simulink library "outp"  (R2021b)
(part 3 of 11)

  bus_selector3/179 -> outpmodule/357(VBCM_WinRROpenedSta_pct)  "<VBCM_WinRROpenedSta_pct>"
  bus_selector13/31 -> outpmodule/953(VTQD_FrUdcMin_V)  "<VTQD_FrUdcMin_V>"
  bus_selector2/16 -> outpmodule/19(VAPM_APSDFLR_cm)  "<VAPM_APSDFLR_cm>"
  outpmodule/782(VOUTP_FDCTHCCREVentZStaSet7_enum) -> bus_creator/782
  bus_selector12/68 -> outpmodule/893(VTPM_ChkStorge_flg)  "<VTPM_ChkStorge_flg>"
  bus_selector3/175 -> outpmodule/353(VBCM_CLWinLockDrStaMem_enum)  "<VBCM_CLWinLockDrStaMem_enum>"
  outpmodule/248(VOUTP_IVIRST_flg) -> bus_creator/248
  bus_selector16/7 -> outpmodule/989(VVMC_VMCCCCtrlAvail_flg)  "<VVMC_VMCCCCtrlAvail_flg>"
  outpmodule/644(VOUTP_ECUGen2_cnt) -> bus_creator/644
  bus_selector11/129 -> outpmodule/778(VTHC_FDCTHCCREVentZStaSet2_enum)  "<VTHC_FDCTHCCREVentZStaSet2_enum>"
  outpmodule/706(VOUTP_FDCTHCREVentZSta_enum) -> bus_creator/706
  bus_selector3/173 -> outpmodule/351(VBCM_PsRWdwReqAP_enum)  "<VBCM_PsRWdwReqAP_enum>"
  bus_selector3/171 -> outpmodule/349(VBCM_PasWdwReqAP_enum)  "<VBCM_PasWdwReqAP_enum>"
  outpmodule/832(VOUTP_LRWheelPress_raw8) -> bus_creator/832
  bus_selector10/35 -> outpmodule/641(VSYS_AcoreRebootCmdACK_flg)  "<VSYS_AcoreRebootCmdACK_flg>"
  bus_selector13/39 -> outpmodule/961(VTQD_EquivAccPedalSWSta_flg)  "<VTQD_EquivAccPedalSWSta_flg>"
  bus_selector3/172 -> outpmodule/350(VBCM_DrRWdwReqAP_enum)  "<VBCM_DrRWdwReqAP_enum>"
  outpmodule/1044(VOUTP_LKAHODDisplayWarning_flg) -> bus_creator/1044
  bus_selector3/170 -> outpmodule/348(VBCM_DrvWdwReqAP_enum)  "<VBCM_DrvWdwReqAP_enum>"
  outpmodule/714(VOUTP_FDCTHCCREVentYSta_enum) -> bus_creator/714
  outpmodule/236(VOUTP_AmbLightBrightness5_enum) -> bus_creator/236
  outpmodule/799(VOUTP_FDCTHCREVentYStaSet5_enum) -> bus_creator/799
  bus_selector3/168 -> outpmodule/346(VBCM_HMIKey8FuncSta_enum)  "<VBCM_HMIKey8FuncSta_enum>"
  bus_selector3/164 -> outpmodule/342(VBCM_HMIKey4FuncSta_enum)  "<VBCM_HMIKey4FuncSta_enum>"
  bus_selector3/165 -> outpmodule/343(VBCM_HMIKey5FuncSta_enum)  "<VBCM_HMIKey5FuncSta_enum>"
  bus_selector3/166 -> outpmodule/344(VBCM_HMIKey6FuncSta_enum)  "<VBCM_HMIKey6FuncSta_enum>"
  outpmodule/1032(VOUTP_RightTurnLightReq_flg) -> bus_creator/1032
  outpmodule/937(VOUTP_FrEDUActTq_Nm) -> bus_creator/937
  outpmodule/178(VOUTP_IVIUserTakeOverAPSSta_flg) -> bus_creator/178
  bus_selector10/3 -> outpmodule/609(VSYS_HWVer3_cnt)  "<VSYS_HWVer3_cnt>"
  bus_selector16/12 -> outpmodule/994(VVMC_LimitPCT_pct)  "<VVMC_LimitPCT_pct>"
  bus_selector3/163 -> outpmodule/341(VBCM_HMIKey3FuncSta_enum)  "<VBCM_HMIKey3FuncSta_enum>"
  outpmodule/788(VOUTP_FDCTHCLEVentYStaSet7_enum) -> bus_creator/788
  bus_selector6/10 -> outpmodule/534(VDKC_DKeyWelcomeSta_enum)  "<VDKC_DKeyWelcomeSta_enum>"
  outpmodule/98(VOUTP_SASSpeedValidTimeOut_flg) -> bus_creator/98
  outpmodule/611(VOUTP_CarModel2_cnt) -> bus_creator/611
  outpmodule/980(VOUTP_ReqOBCIntrV2LEna_enum) -> bus_creator/980
  bus_selector3/158 -> outpmodule/336(VBCM_AutoLockMem_enum)  "<VBCM_AutoLockMem_enum>"
  bus_selector3/160 -> outpmodule/338(VBCM_AutoUnlockMem_enum)  "<VBCM_AutoUnlockMem_enum>"
  outpmodule/892(VOUTP_TPMSStorge_flg) -> bus_creator/892
  bus_selector10/42 -> outpmodule/648(VSYS_Var4_cnt)  "<VSYS_Var4_cnt>"
  outpmodule/491(VOUTP_EngagePFail_flg) -> bus_creator/491
  bus_selector3/157 -> outpmodule/335(VBCM_AutoLockSta_flg)  "<VBCM_AutoLockSta_flg>"
  bus_selector4/138 -> outpmodule/495(VDDM_EDriveSysErrShifterErr_flg)  "<VDDM_EDriveSysErrShifterErr_flg>"
  bus_selector11/83 -> outpmodule/732(VTHC_sigRecircStSet_enum)  "<VTHC_sigRecircStSet_enum>"
  bus_selector3/155 -> outpmodule/333(VBCM_LRightStaCmd_flg)  "<VBCM_LRightStaCmd_flg>"
  outpmodule/999(VOUTP_SafetyCtrl_flg) -> bus_creator/999
  bus_selector3/73 -> outpmodule/251(VBCM_MirrorFlodPos_flg)  "<VBCM_MirrorFlodPos_flg>"
  bus_selector13/25 -> outpmodule/947(VTQD_RgnAbnorSta_flg)  "<VTQD_RgnAbnorSta_flg>"
  bus_selector3/161 -> outpmodule/339(VBCM_HMIKey1FuncSta_enum)  "<VBCM_HMIKey1FuncSta_enum>"
  bus_selector12/72 -> outpmodule/897(VTPM_LRPindi_enum)  "<VTPM_LRPindi_enum>"
  bus_selector4/145 -> outpmodule/502(VDDM_VCURLDoorSta_flg)  "<VDDM_VCURLDoorSta_flg>"
  bus_selector2/166 -> outpmodule/169(VAPM_CAASVMCReqA_flg)  "<VAPM_CAASVMCReqA_flg>"
  bus_selector11/20 -> outpmodule/669(VTHC_BatteryMode_enum)  "<VTHC_BatteryMode_enum>"
  bus_selector3/150 -> outpmodule/328(VBCM_SenstivityPosnCmd_enum)  "<VBCM_SenstivityPosnCmd_enum>"
  outpmodule/617(VOUTP_Minor1_cnt) -> bus_creator/617
  outpmodule/225(VOUTP_WiperFixMode_flg) -> bus_creator/225
  bus_selector9/11 -> outpmodule/569(VPMM_LVPwrSta_flg)  "<VPMM_LVPwrSta_flg>"
  outpmodule/906(VOUTP_WriteChkfinRRID_raw) -> bus_creator/906
  outpmodule/228(VOUTP_AmbLightBreath3_enum) -> bus_creator/228
  bus_selector3/151 -> outpmodule/329(VBCM_TimeGapLevelSta_enum)  "<VBCM_TimeGapLevelSta_enum>"
  outpmodule/993(VOUTP_JerkPCT_pct) -> bus_creator/993
  bus_selector3/148 -> outpmodule/326(VBCM_PTGOpenHeight34_enum)  "<VBCM_PTGOpenHeight34_enum>"
  bus_selector2/24 -> outpmodule/27(VAPM_PASAFML_enum)  "<VAPM_PASAFML_enum>"
  bus_selector3/149 -> outpmodule/327(VBCM_PTGOpenHeight57_enum)  "<VBCM_PTGOpenHeight57_enum>"
  outpmodule/689(VOUTP_ACModeMem_enum) -> bus_creator/689
  bus_selector3/146 -> outpmodule/324(VBCM_PTGUserHeight7_cnt)  "<VBCM_PTGUserHeight7_cnt>"
  bus_selector11/36 -> outpmodule/685(VTHC_sigAmbAirT_C)  "<VTHC_sigAmbAirT_C>"
  bus_selector11/106 -> outpmodule/755(VTHC_LEVentModeStaSet123_enum)  "<VTHC_LEVentModeStaSet123_enum>"
  bus_selector3/78 -> outpmodule/256(VBCM_PasWdwCtrlCmd_pct)  "<VBCM_PasWdwCtrlCmd_pct>"
  outpmodule/187(VOUTP_DrDoorSW_flg) -> bus_creator/187
  outpmodule/1002(VOUTP_ISOAccLimit_mps2) -> bus_creator/1002
  bus_selector3/145 -> outpmodule/323(VBCM_PTGUserHeight5_cnt)  "<VBCM_PTGUserHeight5_cnt>"
  bus_selector2/79 -> outpmodule/82(VAPM_RFPulseCountTimeOut_flg)  "<VAPM_RFPulseCountTimeOut_flg>"
  bus_selector12/2 -> outpmodule/827(VTPM_RFBatWarn_flg)  "<VTPM_RFBatWarn_flg>"
  bus_selector3/143 -> outpmodule/321(VBCM_PTGUserHeight3_cnt)  "<VBCM_PTGUserHeight3_cnt>"
  bus_selector3/144 -> outpmodule/322(VBCM_PTGUserHeight4_cnt)  "<VBCM_PTGUserHeight4_cnt>"
  bus_selector4/118 -> outpmodule/475(VDDM_RRPressIndiDTC_raw32)  "<VDDM_RRPressIndiDTC_raw32>"
  bus_selector3/15 -> outpmodule/193(VBCM_RrChargingDoorCtrl_enum)  "<VBCM_RrChargingDoorCtrl_enum>"
  bus_selector3/13 -> outpmodule/191(VBCM_LockSetting_flg)  "<VBCM_LockSetting_flg>"
  outpmodule/231(VOUTP_AmbLightBreath6_enum) -> bus_creator/231
  bus_selector2/4 -> outpmodule/7(VAPM_FSOffSwTimeOut_flg)  "<VAPM_FSOffSwTimeOut_flg>"
  bus_selector3/12 -> outpmodule/190(VBCM_RRDoorSW_flg)  "<VBCM_RRDoorSW_flg>"
  outpmodule/736(VOUTP_AirIntenZone1MSet3_enum) -> bus_creator/736
  outpmodule/914(VOUTP_FlashS3ID_raw) -> bus_creator/914
  bus_selector3/11 -> outpmodule/189(VBCM_RLDoorSW_flg)  "<VBCM_RLDoorSW_flg>"
  bus_selector3/8 -> outpmodule/186(VBCM_TailgateSW_flg)  "<VBCM_TailgateSW_flg>"
  bus_selector3/35 -> outpmodule/213(VBCM_BCMBuzzerReq_flg)  "<VBCM_BCMBuzzerReq_flg>"
  bus_selector2/111 -> outpmodule/114(VAPM_YawRateVTimeOut_flg)  "<VAPM_YawRateVTimeOut_flg>"
  bus_selector3/10 -> outpmodule/188(VBCM_PsDoorSW_flg)  "<VBCM_PsDoorSW_flg>"
  outpmodule/868(VOUTP_S2ID_raw32) -> bus_creator/868
  outpmodule/81(VOUTP_RFPulseCount_enum) -> bus_creator/81
  outpmodule/84(VOUTP_LRPulseCountTimeOut_flg) -> bus_creator/84
  outpmodule/241(VOUTP_AmbLightColor4_enum) -> bus_creator/241
  outpmodule/1028(VOUTP_ADASShftPosnReqA_flg) -> bus_creator/1028
  outpmodule/442(VOUTP_FCM5CSErrDTC_raw32) -> bus_creator/442
  bus_selector16/22 -> outpmodule/1004(VVMC_ISOJerkLimit_mps3)  "<VVMC_ISOJerkLimit_mps3>"
  outpmodule/724(VOUTP_FDCTHCMPreWPTCHeatSta_enum) -> bus_creator/724
  bus_selector2/125 -> outpmodule/128(VAPM_ESCAPSStaTimeOut_flg)  "<VAPM_ESCAPSStaTimeOut_flg>"
  outpmodule/673(VOUTP_CCUAutoLampSts_flg) -> bus_creator/673
  outpmodule/249(VOUTP_CountAlarm_enum) -> bus_creator/249
  bus_selector9/35 -> outpmodule/593(VPMM_LVSilentChrgReq_flg)  "<VPMM_LVSilentChrgReq_flg>"
  outpmodule/118(VOUTP_LongAccelVTimeOut_flg) -> bus_creator/118
  outpmodule/777(VOUTP_FDCTHCCREVentZStaSet1_enum) -> bus_creator/777
  bus_selector2/126 -> outpmodule/129(VAPM_EPBExtReleaseAvail_flg)  "<VAPM_EPBExtReleaseAvail_flg>"
  outpmodule/701(VOUTP_FDCTHCAirIntZ3Sta_enum) -> bus_creator/701
  bus_selector2/124 -> outpmodule/127(VAPM_ESCAPSSta_enum)  "<VAPM_ESCAPSSta_enum>"
  bus_selector9/26 -> outpmodule/584(VPMM_PwrStaONTOPopReq_flg)  "<VPMM_PwrStaONTOPopReq_flg>"
  bus_selector2/137 -> outpmodule/140(VAPM_AVMparkingexcuteTimeOut_flg)  "<VAPM_AVMparkingexcuteTimeOut_flg>"
  bus_selector3/113 -> outpmodule/291(VBCM_DimSwSta_flg)  "<VBCM_DimSwSta_flg>"
  bus_selector3/177 -> outpmodule/355(VBCM_WinRFOpenedSta_pct)  "<VBCM_WinRFOpenedSta_pct>"
  bus_selector4/46 -> outpmodule/403(VDDM_TailgaSWDTC_raw32)  "<VDDM_TailgaSWDTC_raw32>"
  bus_selector11/120 -> outpmodule/769(VTHC_FDCTHCCLEVentZStaSet5_enum)  "<VTHC_FDCTHCCLEVentZStaSet5_enum>"
  bus_selector3/55 -> outpmodule/233(VBCM_AmbLightBrightness2_enum)  "<VBCM_AmbLightBrightness2_enum>"
  bus_selector2/132 -> outpmodule/135(VAPM_EPBSta_enum)  "<VAPM_EPBSta_enum>"
  bus_selector2/131 -> outpmodule/134(VAPM_EPBErrStaTimeOut_flg)  "<VAPM_EPBErrStaTimeOut_flg>"
  bus_selector4/34 -> outpmodule/391(VDDM_HVRlyOpDTC_raw32)  "<VDDM_HVRlyOpDTC_raw32>"
  bus_selector6/13 -> outpmodule/537(VDKC_UIDLowPowerSta_enum)  "<VDKC_UIDLowPowerSta_enum>"
  bus_selector11/175 -> outpmodule/824(VTHC_THSysErrlampReq_flg)  "<VTHC_THSysErrlampReq_flg>"
  bus_selector6/2 -> outpmodule/526(VDKC_DKCAuthSta_enum)  "<VDKC_DKCAuthSta_enum>"
  bus_selector4/38 -> outpmodule/395(VDDM_LVSupLoDTC_raw32)  "<VDDM_LVSupLoDTC_raw32>"
  outpmodule/56(VOUTP_LFRawWhlSpeedVTimeOut_flg) -> bus_creator/56
  bus_selector11/18 -> outpmodule/667(VTHC_FDRrAPTCHeatPwrCmd_W)  "<VTHC_FDRrAPTCHeatPwrCmd_W>"
  outpmodule/54(VOUTP_RRRawWhlSpeedTimeOut_flg) -> bus_creator/54
  outpmodule/911(VOUTP_Prepresstempvalid_enum) -> bus_creator/911
  outpmodule/217(VOUTP_RoomLampH_flg) -> bus_creator/217
  bus_selector2/162 -> outpmodule/165(VAPM_CAASSta_enum)  "<VAPM_CAASSta_enum>"
  bus_selector11/166 -> outpmodule/815(VTHC_FACESet_enum)  "<VTHC_FACESet_enum>"
  bus_selector3/28 -> outpmodule/206(VBCM_LDRL_flg)  "<VBCM_LDRL_flg>"
  outpmodule/55(VOUTP_LFRawWhlSpeedV_flg) -> bus_creator/55
  outpmodule/252(VOUTP_FuelDoorPos_flg) -> bus_creator/252
  bus_selector11/113 -> outpmodule/762(VTHC_FDCTHCLEVentZStaSet4_enum)  "<VTHC_FDCTHCLEVentZStaSet4_enum>"
  outpmodule/53(VOUTP_RRRawWhlSpeed_kph) -> bus_creator/53
  outpmodule/49(VOUTP_RFRawWhlSpeed_kph) -> bus_creator/49
  outpmodule/641(VOUTP_AcoreRebootCmdACK_flg) -> bus_creator/641
  outpmodule/95(VOUTP_SASSpeed_degps) -> bus_creator/95
  bus_selector2/158 -> outpmodule/161(VAPM_APSExitCondition_enum)  "<VAPM_APSExitCondition_enum>"
  outpmodule/50(VOUTP_RFRawWhlSpeedTimeOut_flg) -> bus_creator/50
  outpmodule/921(VOUTP_ModelVersion_raw) -> bus_creator/921
  outpmodule/734(VOUTP_AirIntenZone1MSet1_enum) -> bus_creator/734
  bus_selector9/23 -> outpmodule/581(VPMM_LowSOCWarn_enum)  "<VPMM_LowSOCWarn_enum>"
  outpmodule/308(VOUTP_RmLpModeENMem_enum) -> bus_creator/308
  outpmodule/48(VOUTP_LFRawWhlSpeedTimeOut_flg) -> bus_creator/48
  outpmodule/1061(VOUTP_ADASLanetypeR_enum) -> bus_creator/1061
  outpmodule/988(VOUTP_VMCACCCtrlAvail_flg) -> bus_creator/988
  bus_selector3/114 -> outpmodule/292(VBCM_PassSWSta_flg)  "<VBCM_PassSWSta_flg>"
  bus_selector4/43 -> outpmodule/400(VDDM_FRDoorSWDTC_raw32)  "<VDDM_FRDoorSWDTC_raw32>"
  outpmodule/524(VOUTP_EAPS2NRM_pct) -> bus_creator/524
  outpmodule/505(VOUTP_VCUHoodSWSta_flg) -> bus_creator/505
  outpmodule/46(VOUTP_BrkPedalPosTimeOut_flg) -> bus_creator/46
  bus_selector11/54 -> outpmodule/703(VTHC_FDCTHCREVentModeSta_enum)  "<VTHC_FDCTHCREVentModeSta_enum>"
  outpmodule/44(VOUTP_ModOperation_enum) -> bus_creator/44
  outpmodule/915(VOUTP_FlashS4ID_raw) -> bus_creator/915
  outpmodule/575(VOUTP_DrSeatSta_enum) -> bus_creator/575
  bus_selector14/1 -> outpmodule/974(VTQR_FrTMTqReq_Nm)  "<VTQR_FrTMTqReq_Nm>"
  outpmodule/42(VOUTP_SNSRLayout_enum) -> bus_creator/42
  outpmodule/262(VOUTP_AmbDimEN_flg) -> bus_creator/262
  outpmodule/40(VOUTP_USSStaFCL_flg) -> bus_creator/40
  bus_selector2/90 -> outpmodule/93(VAPM_SASAngle_Deg)  "<VAPM_SASAngle_Deg>"
  bus_selector3/82 -> outpmodule/260(VBCM_AmbFunEN_flg)  "<VBCM_AmbFunEN_flg>"
  bus_selector16/15 -> outpmodule/997(VVMC_SingleWhlSlipRatioCtrl_flg)  "<VVMC_SingleWhlSlipRatioCtrl_flg>"
  outpmodule/360(VOUTP_C3BMS6LCDTC_raw32) -> bus_creator/360
  outpmodule/749(VOUTP_FDCFGSAirIntStaSet123_enum) -> bus_creator/749
  outpmodule/537(VOUTP_UIDLowPowerSta_enum) -> bus_creator/537
  outpmodule/41(VOUTP_Chime_enum) -> bus_creator/41
  bus_selector2/48 -> outpmodule/51(VAPM_LRRawWhlSpeed_kph)  "<VAPM_LRRawWhlSpeed_kph>"
  bus_selector4/40 -> outpmodule/397(VDDM_DrStSWDTC_raw32)  "<VDDM_DrStSWDTC_raw32>"
  outpmodule/732(VOUTP_sigRecircStSet_enum) -> bus_creator/732
  outpmodule/522(VOUTP_ResetPedalZeroPosStart_flg) -> bus_creator/522
  outpmodule/38(VOUTP_USSStaFLL_flg) -> bus_creator/38
  outpmodule/804(VOUTP_FDCTHCCREVentYStaSet4_enum) -> bus_creator/804
  outpmodule/35(VOUTP_USSStaFMR_flg) -> bus_creator/35
  bus_selector2/77 -> outpmodule/80(VAPM_LFPulseCountTimeOut_flg)  "<VAPM_LFPulseCountTimeOut_flg>"
  outpmodule/109(VOUTP_LongAccel_Gps) -> bus_creator/109
  outpmodule/130(VOUTP_EPBExtReleaseAvailTimeOut_flg) -> bus_creator/130
  outpmodule/36(VOUTP_USSStaFML_flg) -> bus_creator/36
  bus_selector4/31 -> outpmodule/388(VDDM_MidLvSaChkDTC_raw32)  "<VDDM_MidLvSaChkDTC_raw32>"
  bus_selector3/9 -> outpmodule/187(VBCM_DrDoorSW_flg)  "<VBCM_DrDoorSW_flg>"
  outpmodule/33(VOUTP_USSStaRCR_flg) -> bus_creator/33
  outpmodule/858(VOUTP_LRWheelPSW_raw8) -> bus_creator/858
  outpmodule/986(VOUTP_MeterIndSpeed_raw32) -> bus_creator/986
  outpmodule/32(VOUTP_USSStaRLL_flg) -> bus_creator/32
  bus_selector11/35 -> outpmodule/684(VTHC_sigCbnSolarRight_W)  "<VTHC_sigCbnSolarRight_W>"
  outpmodule/34(VOUTP_USSStaRCL_flg) -> bus_creator/34
  outpmodule/474(VOUTP_LRPressIndiDTC_raw32) -> bus_creator/474
  bus_selector13/32 -> outpmodule/954(VTQD_FrUdcMax_V)  "<VTQD_FrUdcMax_V>"
  outpmodule/825(VOUTP_sigCbnPTCPwrAct_W) -> bus_creator/825
  outpmodule/115(VOUTP_LatAccelV_flg) -> bus_creator/115
  outpmodule/31(VOUTP_USSStaRLR_flg) -> bus_creator/31
  outpmodule/955(VOUTP_RrIdcMin_A) -> bus_creator/955
  bus_selector4/70 -> outpmodule/427(VDDM_RMRUSSDTC_raw32)  "<VDDM_RMRUSSDTC_raw32>"
  outpmodule/330(VOUTP_ACCLevelMem12_enum) -> bus_creator/330
  outpmodule/30(VOUTP_USSStaRML_flg) -> bus_creator/30
  bus_selector4/56 -> outpmodule/413(VDDM_ESC1NoComDTC_raw32)  "<VDDM_ESC1NoComDTC_raw32>"
  bus_selector8/8 -> outpmodule/554(VNMM_RptMsgReq_flg)  "<VNMM_RptMsgReq_flg>"
  bus_selector12/78 -> outpmodule/903(VTPM_WriteChkfinLFID_raw)  "<VTPM_WriteChkfinLFID_raw>"
  outpmodule/29(VOUTP_USSStaRMR_flg) -> bus_creator/29
  outpmodule/180(VOUTP_TailgateRemote_enum) -> bus_creator/180
  bus_selector3/22 -> outpmodule/200(VBCM_PosLamp_flg)  "<VBCM_PosLamp_flg>"
  outpmodule/135(VOUTP_EPBSta_enum) -> bus_creator/135
  outpmodule/28(VOUTP_PASAFCR_enum) -> bus_creator/28
  outpmodule/27(VOUTP_PASAFML_enum) -> bus_creator/27
  bus_selector3/147 -> outpmodule/325(VBCM_PTGOpenHeight12_enum)  "<VBCM_PTGOpenHeight12_enum>"
  bus_selector3/32 -> outpmodule/210(VBCM_HazardSW_flg)  "<VBCM_HazardSW_flg>"
  outpmodule/747(VOUTP_FDCFGSChStaSet123_enum) -> bus_creator/747
  outpmodule/112(VOUTP_MCPressureTimeOut_flg) -> bus_creator/112
  outpmodule/216(VOUTP_RrDefog_flg) -> bus_creator/216
  outpmodule/26(VOUTP_PASAFMR_enum) -> bus_creator/26
  outpmodule/25(VOUTP_PASARCL_enum) -> bus_creator/25
  bus_selector3/154 -> outpmodule/332(VBCM_ACCLevelMem57_enum)  "<VBCM_ACCLevelMem57_enum>"
  bus_selector3/61 -> outpmodule/239(VBCM_AmbLightColor2_enum)  "<VBCM_AmbLightColor2_enum>"
  outpmodule/23(VOUTP_PASARML_enum) -> bus_creator/23
  bus_selector4/61 -> outpmodule/418(VDDM_DiagFRTSDTC_raw32)  "<VDDM_DiagFRTSDTC_raw32>"
  outpmodule/564(VOUTP_DCDCEnaReq_flg) -> bus_creator/564
  outpmodule/107(VOUTP_LatAccel_Gps) -> bus_creator/107
  bus_selector3/43 -> outpmodule/221(VBCM_FrWiperL_flg)  "<VBCM_FrWiperL_flg>"
  bus_selector2/2 -> outpmodule/5(VAPM_VehSpeedTimeOut_flg)  "<VAPM_VehSpeedTimeOut_flg>"
  outpmodule/24(VOUTP_PASARCR_enum) -> bus_creator/24
  bus_selector10/8 -> outpmodule/614(VSYS_ECU2_cnt)  "<VSYS_ECU2_cnt>"
  outpmodule/101(VOUTP_SASV_flg) -> bus_creator/101
  outpmodule/144(VOUTP_AVMErrSTATimeOut_flg) -> bus_creator/144
  bus_selector2/128 -> outpmodule/131(VAPM_EPBExtApplyAvail_flg)  "<VAPM_EPBExtApplyAvail_flg>"
  outpmodule/22(VOUTP_PASARMR_enum) -> bus_creator/22
  outpmodule/20(VOUTP_APSDFLL_cm) -> bus_creator/20
  outpmodule/649(VOUTP_Var5_cnt) -> bus_creator/649
  outpmodule/21(VOUTP_PASAFCL_enum) -> bus_creator/21
  bus_selector2/69 -> outpmodule/72(VAPM_LFPulseCountVTimeOut_flg)  "<VAPM_LFPulseCountVTimeOut_flg>"
  outpmodule/19(VOUTP_APSDFLR_cm) -> bus_creator/19
  outpmodule/717(VOUTP_FDCFGSAirIntSta_enum) -> bus_creator/717
  outpmodule/207(VOUTP_RDRL_flg) -> bus_creator/207
  bus_selector10/23 -> outpmodule/629(VSYS_SHA2_cnt)  "<VSYS_SHA2_cnt>"
  outpmodule/18(VOUTP_APSDRLL_cm) -> bus_creator/18
  outpmodule/547(VOUTP_AllCANTxReq_flg) -> bus_creator/547
  bus_selector9/40 -> outpmodule/598(VPMM_CtrlFrEDUINVERTER_flg)  "<VPMM_CtrlFrEDUINVERTER_flg>"
  bus_selector2/134 -> outpmodule/137(VAPM_AVMparkingcancel_enum)  "<VAPM_AVMparkingcancel_enum>"
  bus_selector4/82 -> outpmodule/439(VDDM_FCM4NoComDTC_raw32)  "<VDDM_FCM4NoComDTC_raw32>"
  outpmodule/16(VOUTP_PASDFCL_cm) -> bus_creator/16
  outpmodule/738(VOUTP_AirIntenZone1MSet5_enum) -> bus_creator/738
  bus_selector3/24 -> outpmodule/202(VBCM_HBeam_flg)  "<VBCM_HBeam_flg>"
  outpmodule/226(VOUTP_AmbLightBreath1_enum) -> bus_creator/226
  outpmodule/17(VOUTP_APSDRLR_cm) -> bus_creator/17
  outpmodule/13(VOUTP_PASDFMR_cm) -> bus_creator/13
  bus_selector9/34 -> outpmodule/592(VPMM_LVSilentChrgSta_enum)  "<VPMM_LVSilentChrgSta_enum>"
  bus_selector4/144 -> outpmodule/501(VDDM_VCUFRDoorSta_flg)  "<VDDM_VCUFRDoorSta_flg>"
  outpmodule/14(VOUTP_PASDFML_cm) -> bus_creator/14
  outpmodule/15(VOUTP_PASDFCR_cm) -> bus_creator/15
  outpmodule/728(VOUTP_FaceMSet_enum) -> bus_creator/728
  outpmodule/11(VOUTP_PASDRCR_cm) -> bus_creator/11
  outpmodule/936(VOUTP_DriverWhlTqDemRr_Nm) -> bus_creator/936
  outpmodule/638(VOUTP_FdcSlpTime_sec) -> bus_creator/638
  outpmodule/944(VOUTP_FrEDUAvailBrkRgnTqV_flg) -> bus_creator/944
  bus_selector2/171 -> outpmodule/174(VAPM_RAPSBCMLockReq_flg)  "<VAPM_RAPSBCMLockReq_flg>"
  bus_selector4/128 -> outpmodule/485(VDDM_5vAPS1PwrErrDTC_raw32)  "<VDDM_5vAPS1PwrErrDTC_raw32>"
  outpmodule/407(VOUTP_APS2SigOoRDTC_raw32) -> bus_creator/407
  outpmodule/12(VOUTP_PASDRCL_cm) -> bus_creator/12
  bus_selector11/164 -> outpmodule/813(VTHC_ACModeSet123_enum)  "<VTHC_ACModeSet123_enum>"
  bus_selector11/51 -> outpmodule/700(VTHC_sigDfrstSt_flg)  "<VTHC_sigDfrstSt_flg>"
  outpmodule/140(VOUTP_AVMparkingexcuteTimeOut_flg) -> bus_creator/140
  bus_selector8/7 -> outpmodule/553(VNMM_PNI_flg)  "<VNMM_PNI_flg>"
  outpmodule/191(VOUTP_LockSetting_flg) -> bus_creator/191
  outpmodule/9(VOUTP_PASDRMR_cm) -> bus_creator/9
  bus_selector13/36 -> outpmodule/958(VTQD_RrUdcMax_V)  "<VTQD_RrUdcMax_V>"
  outpmodule/7(VOUTP_FSOffSwTimeOut_flg) -> bus_creator/7
  bus_selector2/55 -> outpmodule/58(VAPM_RFRawWhlSpeedVTimeOut_flg)  "<VAPM_RFRawWhlSpeedVTimeOut_flg>"
  outpmodule/224(VOUTP_WasherCtrl_enum) -> bus_creator/224
  outpmodule/5(VOUTP_VehSpeedTimeOut_flg) -> bus_creator/5
  outpmodule/504(VOUTP_SysAllowReadySta_flg) -> bus_creator/504
  outpmodule/3(VOUTP_VehHVPwrAvail4THCM_W) -> bus_creator/3
  bus_selector9/43 -> outpmodule/601(VPMM_PwrStaTOSta_enum)  "<VPMM_PwrStaTOSta_enum>"
  outpmodule/912(VOUTP_FlashS1ID_raw) -> bus_creator/912
  outpmodule/4(VOUTP_VehSpeed_kph) -> bus_creator/4
  bus_selector3/156 -> outpmodule/334(VBCM_LLeftStaCmd_flg)  "<VBCM_LLeftStaCmd_flg>"
  bus_selector10/9 -> outpmodule/615(VSYS_Major1_cnt)  "<VSYS_Major1_cnt>"
  bus_selector3/66 -> outpmodule/244(VBCM_LampPwr_flg)  "<VBCM_LampPwr_flg>"
  bus_selector10/33 -> outpmodule/639(VSYS_PmicBootReason_enum)  "<VSYS_PmicBootReason_enum>"
  outpmodule/2(VOUTP_LVBattVoltSta_enum) -> bus_creator/2
  bus_selector16/4 -> outpmodule/986(VVMC_MeterIndSpeed_raw32)  "<VVMC_MeterIndSpeed_raw32>"
  outpmodule/1(VOUTP_HVTHCMSysAvail_enum) -> bus_creator/1
  outpmodule/59(VOUTP_LRRawWhlSpeedV_flg) -> bus_creator/59
  bus_selector3/4 -> outpmodule/182(VBCM_AllDoorSW_flg)  "<VBCM_AllDoorSW_flg>"
  outpmodule/58(VOUTP_RFRawWhlSpeedVTimeOut_flg) -> bus_creator/58
  outpmodule/170(VOUTP_APSShiftPosnReq_enum) -> bus_creator/170
  bus_selector4/28 -> outpmodule/385(VDDM_BMSRdyDTC_raw32)  "<VDDM_BMSRdyDTC_raw32>"
  bus_selector12/41 -> outpmodule/866(VTPM_RRSensorMode_flg)  "<VTPM_RRSensorMode_flg>"
  bus_selector11/22 -> outpmodule/671(VTHC_CabinMode_enum)  "<VTHC_CabinMode_enum>"
  outpmodule/167(VOUTP_DKCParkingModeCmd_enum) -> bus_creator/167
  outpmodule/884(VOUTP_S3WheelDebugALTU_pct) -> bus_creator/884
  outpmodule/1047(VOUTP_ADASLaneModeL_enum) -> bus_creator/1047
  outpmodule/82(VOUTP_RFPulseCountTimeOut_flg) -> bus_creator/82
  outpmodule/52(VOUTP_LRRawWhlSpeedTimeOut_flg) -> bus_creator/52
  outpmodule/776(VOUTP_FDCTHCREVentZStaSet7_enum) -> bus_creator/776
  outpmodule/165(VOUTP_CAASSta_enum) -> bus_creator/165
  outpmodule/162(VOUTP_APSAngleTarget_Deg) -> bus_creator/162
  bus_selector10/30 -> outpmodule/636(VSYS_NvWriteReqRisingEdge_flg)  "<VSYS_NvWriteReqRisingEdge_flg>"
  bus_selector6/3 -> outpmodule/527(VDKC_TimeSNDKCFbk_cnt)  "<VDKC_TimeSNDKCFbk_cnt>"
  outpmodule/210(VOUTP_HazardSW_flg) -> bus_creator/210
  outpmodule/161(VOUTP_APSExitCondition_enum) -> bus_creator/161
  outpmodule/784(VOUTP_FDCTHCLEVentYStaSet2_enum) -> bus_creator/784
  outpmodule/159(VOUTP_APSSWVer_enum) -> bus_creator/159
  outpmodule/854(VOUTP_RFWheelTmpIndi_flg) -> bus_creator/854
  bus_selector11/119 -> outpmodule/768(VTHC_FDCTHCCLEVentZStaSet4_enum)  "<VTHC_FDCTHCCLEVentZStaSet4_enum>"
  outpmodule/160(VOUTP_APSHWVer_enum) -> bus_creator/160
  bus_selector9/31 -> outpmodule/589(VPMM_TimerAllowSleep_flg)  "<VPMM_TimerAllowSleep_flg>"
  bus_selector10/11 -> outpmodule/617(VSYS_Minor1_cnt)  "<VSYS_Minor1_cnt>"
  outpmodule/205(VOUTP_ReverseLamp_flg) -> bus_creator/205
  bus_selector4/14 -> outpmodule/371(VDDM_C1ABM1CSDTC_raw32)  "<VDDM_C1ABM1CSDTC_raw32>"
  outpmodule/157(VOUTP_APSProgressPCT_pct) -> bus_creator/157
  outpmodule/158(VOUTP_APSRQDisplay_enum) -> bus_creator/158
  bus_selector10/22 -> outpmodule/628(VSYS_SHA1_cnt)  "<VSYS_SHA1_cnt>"
  bus_selector4/146 -> outpmodule/503(VDDM_VCURRDoorSta_flg)  "<VDDM_VCURRDoorSta_flg>"
  bus_selector4/21 -> outpmodule/378(VDDM_BrkSWNoBacDTC_raw32)  "<VDDM_BrkSWNoBacDTC_raw32>"
  outpmodule/984(VOUTP_VehicleSpeed_mph) -> bus_creator/984
  outpmodule/156(VOUTP_DriverSeatBeltCmdTimeOut_flg) -> bus_creator/156
  outpmodule/145(VOUTP_IVIStatus_flg) -> bus_creator/145
  outpmodule/155(VOUTP_DriverSeatBeltCmd_flg) -> bus_creator/155
  outpmodule/833(VOUTP_RRWheelPress_raw8) -> bus_creator/833
  bus_selector2/57 -> outpmodule/60(VAPM_LRRawWhlSpeedVTimeOut_flg)  "<VAPM_LRRawWhlSpeedVTimeOut_flg>"
  outpmodule/154(VOUTP_TCSActiveTimeOut_flg) -> bus_creator/154
  bus_selector3/20 -> outpmodule/198(VBCM_Dimmer_pct)  "<VBCM_Dimmer_pct>"
  bus_selector16/29 -> outpmodule/1011(VVMC_LKAStrToqReq_Nm)  "<VVMC_LKAStrToqReq_Nm>"
  bus_selector3/52 -> outpmodule/230(VBCM_AmbLightBreath5_enum)  "<VBCM_AmbLightBreath5_enum>"
  outpmodule/153(VOUTP_TCSActive_flg) -> bus_creator/153
  bus_selector16/16 -> outpmodule/998(VVMC_LatAccCtrl_flg)  "<VVMC_LatAccCtrl_flg>"
  outpmodule/917(VOUTP_WritingCnt_enum) -> bus_creator/917
  outpmodule/363(VOUTP_C3BMS1LCDTC_raw32) -> bus_creator/363
  outpmodule/639(VOUTP_PmicBootReason_enum) -> bus_creator/639
  bus_selector2/85 -> outpmodule/88(VAPM_ShifterHandleCmdTimeOut_flg)  "<VAPM_ShifterHandleCmdTimeOut_flg>"
  bus_selector2/123 -> outpmodule/126(VAPM_ESCStandstillTimeOut_flg)  "<VAPM_ESCStandstillTimeOut_flg>"
  outpmodule/152(VOUTP_ABSActiveTimeOut_flg) -> bus_creator/152
  bus_selector11/24 -> outpmodule/673(VTHC_CCUAutoLampSts_flg)  "<VTHC_CCUAutoLampSts_flg>"
  outpmodule/151(VOUTP_ABSActive_flg) -> bus_creator/151
  outpmodule/113(VOUTP_YawRateV_flg) -> bus_creator/113
  bus_selector16/24 -> outpmodule/1006(VVMC_DISCReqAcc_mps2)  "<VVMC_DISCReqAcc_mps2>"
  outpmodule/172(VOUTP_APSVMCReqA_flg) -> bus_creator/172
  outpmodule/171(VOUTP_APSSpeedCMD_kph) -> bus_creator/171
  bus_selector3/44 -> outpmodule/222(VBCM_FrWiperH_flg)  "<VBCM_FrWiperH_flg>"
  bus_selector15/7 -> outpmodule/982(VV2L_HVPO120VGrpBLDSt_enum)  "<VV2L_HVPO120VGrpBLDSt_enum>"
  bus_selector9/37 -> outpmodule/595(VPMM_CtrlFrPwrStbA1P_flg)  "<VPMM_CtrlFrPwrStbA1P_flg>"
  outpmodule/652(VOUTP_FDSOV2Cmd_flg) -> bus_creator/652
  outpmodule/950(VOUTP_RrRgnPermSta_flg) -> bus_creator/950
  outpmodule/663(VOUTP_FDEWP2Cmd_enum) -> bus_creator/663
  bus_selector4/122 -> outpmodule/479(VDDM_RRWheelTmpHighDTC_raw32)  "<VDDM_RRWheelTmpHighDTC_raw32>"
  outpmodule/60(VOUTP_LRRawWhlSpeedVTimeOut_flg) -> bus_creator/60
  bus_selector14/2 -> outpmodule/975(VTQR_RrTMTqReq_Nm)  "<VTQR_RrTMTqReq_Nm>"
  bus_selector11/162 -> outpmodule/811(VTHC_SettempZon1Set5_enum)  "<VTHC_SettempZon1Set5_enum>"
  bus_selector11/68 -> outpmodule/717(VTHC_FDCFGSAirIntSta_enum)  "<VTHC_FDCFGSAirIntSta_enum>"
  bus_selector2/129 -> outpmodule/132(VAPM_EPBExtApplyAvailTimeOut_flg)  "<VAPM_EPBExtApplyAvailTimeOut_flg>"
  bus_selector3/60 -> outpmodule/238(VBCM_AmbLightColor1_enum)  "<VBCM_AmbLightColor1_enum>"
  outpmodule/77(VOUTP_RRPulseCountV_flg) -> bus_creator/77
  outpmodule/75(VOUTP_LRPulseCountV_flg) -> bus_creator/75
  bus_selector4/125 -> outpmodule/482(VDDM_LRSensorFailDTC_raw32)  "<VDDM_LRSensorFailDTC_raw32>"
  outpmodule/80(VOUTP_LFPulseCountTimeOut_flg) -> bus_creator/80
  outpmodule/74(VOUTP_RFPulseCountVTimeOut_flg) -> bus_creator/74
  bus_selector3/174 -> outpmodule/352(VBCM_CLWinLockDrSta_flg)  "<VBCM_CLWinLockDrSta_flg>"
  bus_selector4/37 -> outpmodule/394(VDDM_IniLVLoDTC_raw32)  "<VDDM_IniLVLoDTC_raw32>"
  outpmodule/540(VOUTP_KeyNumSta_enum) -> bus_creator/540
  outpmodule/73(VOUTP_RFPulseCountV_flg) -> bus_creator/73
  outpmodule/72(VOUTP_LFPulseCountVTimeOut_flg) -> bus_creator/72
  outpmodule/973(VOUTP_SetSpdLimWarn_flg) -> bus_creator/973
  bus_selector9/41 -> outpmodule/599(VPMM_HWResetSta_enum)  "<VPMM_HWResetSta_enum>"
  bus_selector11/23 -> outpmodule/672(VTHC_CCUACLampSts_flg)  "<VTHC_CCUACLampSts_flg>"
  outpmodule/956(VOUTP_RrIdcMax_A) -> bus_creator/956
  outpmodule/71(VOUTP_LFPulseCountV_flg) -> bus_creator/71
  outpmodule/43(VOUTP_StaFSya_flg) -> bus_creator/43
  outpmodule/773(VOUTP_FDCTHCREVentZStaSet3_enum) -> bus_creator/773
  outpmodule/70(VOUTP_RRWhlRotDirTimeOut_flg) -> bus_creator/70
  bus_selector12/70 -> outpmodule/895(VTPM_LFPindi_enum)  "<VTPM_LFPindi_enum>"
  outpmodule/946(VOUTP_RrEDUAvailBrkRgnTqV_flg) -> bus_creator/946
  bus_selector2/62 -> outpmodule/65(VAPM_RFWhlRotDir_enum)  "<VAPM_RFWhlRotDir_enum>"
  bus_selector15/2 -> outpmodule/977(VV2L_ReqV2LIVIPopup_enum)  "<VV2L_ReqV2LIVIPopup_enum>"
  outpmodule/352(VOUTP_CLWinLockDrSta_flg) -> bus_creator/352
  outpmodule/117(VOUTP_LongAccelV_flg) -> bus_creator/117
  bus_selector11/140 -> outpmodule/789(VTHC_FDCTHCCLEVentYStaSet1_enum)  "<VTHC_FDCTHCCLEVentYStaSet1_enum>"
  outpmodule/68(VOUTP_LRWhlRotDirTimeOut_flg) -> bus_creator/68
  outpmodule/844(VOUTP_RFWheelDebug_flg) -> bus_creator/844
  outpmodule/67(VOUTP_LRWhlRotDir_enum) -> bus_creator/67
  bus_selector16/17 -> outpmodule/999(VVMC_SafetyCtrl_flg)  "<VVMC_SafetyCtrl_flg>"
  bus_selector13/49 -> outpmodule/971(VTQD_VehActSpd_kph)  "<VTQD_VehActSpd_kph>"
  bus_selector11/61 -> outpmodule/710(VTHC_FDCTHCCLEVentYSta_enum)  "<VTHC_FDCTHCCLEVentYSta_enum>"
  outpmodule/105(VOUTP_YawRate_degps) -> bus_creator/105
  outpmodule/1056(VOUTP_LVDAFailinfo_flg) -> bus_creator/1056
  bus_selector16/6 -> outpmodule/988(VVMC_VMCACCCtrlAvail_flg)  "<VVMC_VMCACCCtrlAvail_flg>"
  bus_selector13/44 -> outpmodule/966(VTQD_SaveRegenMode_enum)  "<VTQD_SaveRegenMode_enum>"
  outpmodule/66(VOUTP_RFWhlRotDirTimeOut_flg) -> bus_creator/66
  outpmodule/677(VOUTP_sigWindDirZon1St_enum) -> bus_creator/677
  bus_selector4/101 -> outpmodule/458(VDDM_Shifter1RCErrDTC_raw32)  "<VDDM_Shifter1RCErrDTC_raw32>"
  outpmodule/196(VOUTP_DoorLockIND_flg) -> bus_creator/196
  outpmodule/960(VOUTP_CreepON_flg) -> bus_creator/960
  outpmodule/365(VOUTP_C3CCU1CSDTC_raw32) -> bus_creator/365
  outpmodule/637(VOUTP_FdcSlpReqRisingEdge_flg) -> bus_creator/637
  outpmodule/96(VOUTP_SASSpeedTimeOut_flg) -> bus_creator/96
  outpmodule/65(VOUTP_RFWhlRotDir_enum) -> bus_creator/65
  outpmodule/188(VOUTP_PsDoorSW_flg) -> bus_creator/188
  outpmodule/64(VOUTP_LFWhlRotDirTimeOut_flg) -> bus_creator/64
  outpmodule/688(VOUTP_FDRecyAutoCmd_enum) -> bus_creator/688
  outpmodule/124(VOUTP_BrkSwVTimeOut_flg) -> bus_creator/124
  bus_selector11/11 -> outpmodule/660(VTHC_CoolgFanActDuty_pct)  "<VTHC_CoolgFanActDuty_pct>"
  bus_selector11/118 -> outpmodule/767(VTHC_FDCTHCCLEVentZStaSet3_enum)  "<VTHC_FDCTHCCLEVentZStaSet3_enum>"
  bus_selector9/18 -> outpmodule/576(VPMM_PwrStaSelect_enum)  "<VPMM_PwrStaSelect_enum>"
  outpmodule/10(VOUTP_PASDRML_cm) -> bus_creator/10
  outpmodule/285(VOUTP_AmbBrightnessSta2_enum) -> bus_creator/285
  outpmodule/62(VOUTP_RRRawWhlSpeedVTimeOut_flg) -> bus_creator/62
  bus_selector4/119 -> outpmodule/476(VDDM_LFWheelTmpHighDTC_raw32)  "<VDDM_LFWheelTmpHighDTC_raw32>"
  bus_selector3/169 -> outpmodule/347(VBCM_AutoWipHSpdENSta_flg)  "<VBCM_AutoWipHSpdENSta_flg>"
  outpmodule/61(VOUTP_RRRawWhlSpeedV_flg) -> bus_creator/61
  outpmodule/544(VOUTP_DISCTargetSpd_kph) -> bus_creator/544
  bus_selector11/60 -> outpmodule/709(VTHC_FDCTHCLVentENSta_flg)  "<VTHC_FDCTHCLVentENSta_flg>"
  bus_selector4/44 -> outpmodule/401(VDDM_RRDoorSWDTC_raw32)  "<VDDM_RRDoorSWDTC_raw32>"
  bus_selector16/114 -> outpmodule/1096(VVMC_FDCVMCMaxAngCtrlOutTqLim_Nm)  "<VVMC_FDCVMCMaxAngCtrlOutTqLim_Nm>"
  outpmodule/751(VOUTP_LVentENSet_enum) -> bus_creator/751
  bus_selector11/152 -> outpmodule/801(VTHC_FDCTHCCREVentYStaSet1_enum)  "<VTHC_FDCTHCCREVentYStaSet1_enum>"
  bus_selector11/9 -> outpmodule/658(VTHC_FDTWVCmd_pct)  "<VTHC_FDTWVCmd_pct>"
  outpmodule/1000(VOUTP_SPD2ACCAct_flg) -> bus_creator/1000
  bus_selector16/115 -> outpmodule/1097(VVMC_FDCVMCDrInpTqBstGn_pct)  "<VVMC_FDCVMCDrInpTqBstGn_pct>"
  outpmodule/47(VOUTP_LFRawWhlSpeed_kph) -> bus_creator/47
  outpmodule/461(VOUTP_ESC7CSErrDTC_raw32) -> bus_creator/461
  bus_selector16/113 -> outpmodule/1095(VVMC_FDCVMCDrInpTqBstAct_flg)  "<VVMC_FDCVMCDrInpTqBstAct_flg>"
  bus_selector16/112 -> outpmodule/1094(VVMC_FDCVMCAngCtrlTqWtGn_pct)  "<VVMC_FDCVMCAngCtrlTqWtGn_pct>"
  outpmodule/703(VOUTP_FDCTHCREVentModeSta_enum) -> bus_creator/703
  outpmodule/202(VOUTP_HBeam_flg) -> bus_creator/202
  bus_selector16/109 -> outpmodule/1091(VVMC_FDCVMCAPSVRqEPSCtrl_flg)  "<VVMC_FDCVMCAPSVRqEPSCtrl_flg>"
  bus_selector3/153 -> outpmodule/331(VBCM_ACCLevelMem34_enum)  "<VBCM_ACCLevelMem34_enum>"
  outpmodule/438(VOUTP_FCM3CSErrDTC_raw32) -> bus_creator/438
  bus_selector2/20 -> outpmodule/23(VAPM_PASARML_enum)  "<VAPM_PASARML_enum>"
  bus_selector16/110 -> outpmodule/1092(VVMC_FDCVMCAPSAngleTarget_deg)  "<VVMC_FDCVMCAPSAngleTarget_deg>"
  bus_selector11/75 -> outpmodule/724(VTHC_FDCTHCMPreWPTCHeatSta_enum)  "<VTHC_FDCTHCMPreWPTCHeatSta_enum>"
  outpmodule/691(VOUTP_Foot_flg) -> bus_creator/691
  outpmodule/212(VOUTP_RTurnLP_flg) -> bus_creator/212
  bus_selector16/108 -> outpmodule/1090(VVMC_CalibratedGyroZ_Dps)  "<VVMC_CalibratedGyroZ_Dps>"
  bus_selector3/45 -> outpmodule/223(VBCM_RrWiper_flg)  "<VBCM_RrWiper_flg>"
  outpmodule/6(VOUTP_FSOffSw_enum) -> bus_creator/6
  BVMC_outputs/1 -> bus_selector16/1
  outpmodule/710(VOUTP_FDCTHCCLEVentYSta_enum) -> bus_creator/710
  outpmodule/527(VOUTP_TimeSNDKCFbk_cnt) -> bus_creator/527
  outpmodule/142(VOUTP_AVMParkingmodeTimeOut_flg) -> bus_creator/142
  bus_selector3/129 -> outpmodule/307(VBCM_WalkOutLkENMem_enum)  "<VBCM_WalkOutLkENMem_enum>"
  bus_selector16/111 -> outpmodule/1093(VVMC_FDCVMCAPSRqEPSCtrl_flg)  "<VVMC_FDCVMCAPSRqEPSCtrl_flg>"
  bus_selector2/136 -> outpmodule/139(VAPM_AVMparkingexcute_enum)  "<VAPM_AVMparkingexcute_enum>"
  bus_selector2/6 -> outpmodule/9(VAPM_PASDRMR_cm)  "<VAPM_PASDRMR_cm>"
  bus_selector12/49 -> outpmodule/874(VTPM_S4L_enum)  "<VTPM_S4L_enum>"
  outpmodule/1048(VOUTP_ADASLaneModeR_enum) -> bus_creator/1048
  outpmodule/266(VOUTP_AmbColorSta_enum) -> bus_creator/266
  outpmodule/99(VOUTP_SASCAL_flg) -> bus_creator/99
  outpmodule/514(VOUTP_CAN2BusOffDTC_raw32) -> bus_creator/514
  bus_selector16/107 -> outpmodule/1089(VVMC_CalibratedGyroY_Dps)  "<VVMC_CalibratedGyroY_Dps>"
  bus_selector16/106 -> outpmodule/1088(VVMC_CalibratedGyroX_Dps)  "<VVMC_CalibratedGyroX_Dps>"
  outpmodule/164(VOUTP_APSRqEPASCtrl_flg) -> bus_creator/164
  bus_selector2/84 -> outpmodule/87(VAPM_ShifterHandleCmd_enum)  "<VAPM_ShifterHandleCmd_enum>"
  outpmodule/326(VOUTP_PTGOpenHeight34_enum) -> bus_creator/326
  bus_selector16/104 -> outpmodule/1086(VVMC_CalibratedAccY_G)  "<VVMC_CalibratedAccY_G>"
  outpmodule/820(VOUTP_RVentEN_flg) -> bus_creator/820
  bus_selector12/37 -> outpmodule/862(VTPM_AutoLTips_enum)  "<VTPM_AutoLTips_enum>"
  bus_selector2/167 -> outpmodule/170(VAPM_APSShiftPosnReq_enum)  "<VAPM_APSShiftPosnReq_enum>"
  outpmodule/166(VOUTP_DKCPDkeyAreaRAPSSta_enum) -> bus_creator/166
  bus_selector16/103 -> outpmodule/1085(VVMC_CalibratedAccX_G)  "<VVMC_CalibratedAccX_G>"
  bus_selector16/105 -> outpmodule/1087(VVMC_CalibratedAccZ_G)  "<VVMC_CalibratedAccZ_G>"
  bus_selector10/7 -> outpmodule/613(VSYS_ECU1_cnt)  "<VSYS_ECU1_cnt>"
  bus_selector16/99 -> outpmodule/1081(VVMC_IMUEnaCmd_flg)  "<VVMC_IMUEnaCmd_flg>"
  bus_selector3/121 -> outpmodule/299(VBCM_OutMode_enum)  "<VBCM_OutMode_enum>"
  outpmodule/507(VOUTP_CAN1BusErrorDTC_raw32) -> bus_creator/507
  bus_selector16/100 -> outpmodule/1082(VVMC_CAASCtrlAvail_flg)  "<VVMC_CAASCtrlAvail_flg>"
  bus_selector3/64 -> outpmodule/242(VBCM_AmbLightColor5_enum)  "<VBCM_AmbLightColor5_enum>"
  bus_selector16/102 -> outpmodule/1084(VVMC_ExtraMSACtrlSta_enum)  "<VVMC_ExtraMSACtrlSta_enum>"
  bus_selector10/31 -> outpmodule/637(VSYS_FdcSlpReqRisingEdge_flg)  "<VSYS_FdcSlpReqRisingEdge_flg>"
  bus_selector15/1 -> outpmodule/976(VV2L_ReqOBCV2LEna_enum)  "<VV2L_ReqOBCV2LEna_enum>"
  bus_selector16/101 -> outpmodule/1083(VVMC_CAASActive_flg)  "<VVMC_CAASActive_flg>"
  bus_selector16/97 -> outpmodule/1079(VVMC_LongAcc_Gps)  "<VVMC_LongAcc_Gps>"
  bus_selector16/98 -> outpmodule/1080(VVMC_CCMSASpdWar_flg)  "<VVMC_CCMSASpdWar_flg>"
  outpmodule/811(VOUTP_SettempZon1Set5_enum) -> bus_creator/811
  outpmodule/183(VOUTP_BCMDoorLockSta_flg) -> bus_creator/183
  bus_selector16/94 -> outpmodule/1076(VVMC_APSDecReqA_flg)  "<VVMC_APSDecReqA_flg>"
  bus_selector16/95 -> outpmodule/1077(VVMC_APSDecReq_mps2)  "<VVMC_APSDecReq_mps2>"
  bus_selector16/96 -> outpmodule/1078(VVMC_APSReq_enum)  "<VVMC_APSReq_enum>"
  bus_selector16/92 -> outpmodule/1074(VVMC_APSActive_flg)  "<VVMC_APSActive_flg>"
  bus_selector3/38 -> outpmodule/216(VBCM_RrDefog_flg)  "<VBCM_RrDefog_flg>"
  bus_selector3/142 -> outpmodule/320(VBCM_PTGUserHeight2_cnt)  "<VBCM_PTGUserHeight2_cnt>"
  bus_selector16/91 -> outpmodule/1073(VVMC_APSCtrlAvail_flg)  "<VVMC_APSCtrlAvail_flg>"
  bus_selector3/162 -> outpmodule/340(VBCM_HMIKey2FuncSta_enum)  "<VBCM_HMIKey2FuncSta_enum>"
  outpmodule/883(VOUTP_S2WheelDebugALTU_pct) -> bus_creator/883
  bus_selector11/160 -> outpmodule/809(VTHC_SettempZon1Set3_enum)  "<VTHC_SettempZon1Set3_enum>"
  outpmodule/219(VOUTP_TrunkRel_flg) -> bus_creator/219
  bus_selector16/93 -> outpmodule/1075(VVMC_APSStaSys_enum)  "<VVMC_APSStaSys_enum>"
  bus_selector3/128 -> outpmodule/306(VBCM_WalkInUnLkENMem_enum)  "<VBCM_WalkInUnLkENMem_enum>"
  bus_selector16/90 -> outpmodule/1072(VVMC_MSACtrlSta_enum)  "<VVMC_MSACtrlSta_enum>"
  bus_selector6/4 -> outpmodule/528(VDKC_KeyMissSta_flg)  "<VDKC_KeyMissSta_flg>"
  bus_selector16/89 -> outpmodule/1071(VVMC_CCCtrlSta_enum)  "<VVMC_CCCtrlSta_enum>"
  bus_selector16/87 -> outpmodule/1069(VVMC_ACCPedalOvrd_flg)  "<VVMC_ACCPedalOvrd_flg>"
  outpmodule/669(VOUTP_BatteryMode_enum) -> bus_creator/669
  bus_selector16/86 -> outpmodule/1068(VVMC_ACCCtrlAvail_flg)  "<VVMC_ACCCtrlAvail_flg>"
  outpmodule/276(VOUTP_AmbPwrWarnENFlash_enum) -> bus_creator/276
  bus_selector3/53 -> outpmodule/231(VBCM_AmbLightBreath6_enum)  "<VBCM_AmbLightBreath6_enum>"
  outpmodule/94(VOUTP_SASAngleTimeOut_flg) -> bus_creator/94
  outpmodule/552(VOUTP_NodeID_enum) -> bus_creator/552
  outpmodule/932(VOUTP_RrActvDmpDisabReq_flg) -> bus_creator/932
  outpmodule/827(VOUTP_RFBatWarn_flg) -> bus_creator/827
  bus_selector16/85 -> outpmodule/1067(VVMC_FCMLDWFault_flg)  "<VVMC_FCMLDWFault_flg>"
  bus_selector16/84 -> outpmodule/1066(VVMC_FCMLDWRequest_enum)  "<VVMC_FCMLDWRequest_enum>"
  bus_selector3/33 -> outpmodule/211(VBCM_LTurnLP_flg)  "<VBCM_LTurnLP_flg>"
  bus_selector11/137 -> outpmodule/786(VTHC_FDCTHCLEVentYStaSet4_enum)  "<VTHC_FDCTHCLEVentYStaSet4_enum>"
  bus_selector2/135 -> outpmodule/138(VAPM_AVMparkingcancelTimeOut_flg)  "<VAPM_AVMparkingcancelTimeOut_flg>"
  bus_selector16/81 -> outpmodule/1063(VVMC_ADASLanecurveL_raw32)  "<VVMC_ADASLanecurveL_raw32>"
  outpmodule/428(VOUTP_RCRUSSDTC_raw32) -> bus_creator/428
  bus_selector16/82 -> outpmodule/1064(VVMC_ADASLanecurveR_raw32)  "<VVMC_ADASLanecurveR_raw32>"
  bus_selector4/15 -> outpmodule/372(VDDM_C1ABM1LCDTC_raw32)  "<VDDM_C1ABM1LCDTC_raw32>"
  outpmodule/143(VOUTP_AVMErrSTA_flg) -> bus_creator/143
  bus_selector2/91 -> outpmodule/94(VAPM_SASAngleTimeOut_flg)  "<VAPM_SASAngleTimeOut_flg>"
  outpmodule/848(VOUTP_LFPressIndi_enum) -> bus_creator/848
  bus_selector11/67 -> outpmodule/716(VTHC_FDCTHCMAPTCForceOFFSta_flg)  "<VTHC_FDCTHCMAPTCForceOFFSta_flg>"
  bus_selector16/83 -> outpmodule/1065(VVMC_ADASAEBSta_enum)  "<VVMC_ADASAEBSta_enum>"
  outpmodule/395(VOUTP_LVSupLoDTC_raw32) -> bus_creator/395
  bus_selector16/80 -> outpmodule/1062(VVMC_ADASLanetypeL_enum)  "<VVMC_ADASLanetypeL_enum>"
  bus_selector16/78 -> outpmodule/1060(VVMC_FCMACCmode_enum)  "<VVMC_FCMACCmode_enum>"
  bus_selector12/35 -> outpmodule/860(VTPM_RRWheelPSW_raw8)  "<VTPM_RRWheelPSW_raw8>"
  outpmodule/133(VOUTP_EPBErrSta_enum) -> bus_creator/133
  BPMM_outputs/1 -> bus_selector9/1
  outpmodule/87(VOUTP_ShifterHandleCmd_enum) -> bus_creator/87
  bus_selector16/76 -> outpmodule/1058(VVMC_LVDAACCStatusInformation_flg)  "<VVMC_LVDAACCStatusInformation_flg>"
  bus_selector4/143 -> outpmodule/500(VDDM_VCUFLDoorSta_flg)  "<VDDM_VCUFLDoorSta_flg>"
  bus_selector12/36 -> outpmodule/861(VTPM_CWheelTips_enum)  "<VTPM_CWheelTips_enum>"
  outpmodule/899(VOUTP_WriteChkLFID_raw) -> bus_creator/899
  bus_selector16/75 -> outpmodule/1057(VVMC_LVDAWarning_flg)  "<VVMC_LVDAWarning_flg>"
  bus_selector4/22 -> outpmodule/379(VDDM_KeyAuthDTC_raw32)  "<VDDM_KeyAuthDTC_raw32>"
  bus_selector3/91 -> outpmodule/269(VBCM_ATCtrl_enum)  "<VBCM_ATCtrl_enum>"
  outpmodule/51(VOUTP_LRRawWhlSpeed_kph) -> bus_creator/51
  outpmodule/648(VOUTP_Var4_cnt) -> bus_creator/648
  bus_selector16/69 -> outpmodule/1051(VVMC_ADASLDWMute_flg)  "<VVMC_ADASLDWMute_flg>"
  bus_selector16/66 -> outpmodule/1048(VVMC_ADASLaneModeR_enum)  "<VVMC_ADASLaneModeR_enum>"
  bus_selector4/41 -> outpmodule/398(VDDM_FLDoorSWDTC_raw32)  "<VDDM_FLDoorSWDTC_raw32>"
  bus_selector16/68 -> outpmodule/1050(VVMC_ADASISASta_enum)  "<VVMC_ADASISASta_enum>"
  bus_selector16/65 -> outpmodule/1047(VVMC_ADASLaneModeL_enum)  "<VVMC_ADASLaneModeL_enum>"
  outpmodule/69(VOUTP_RRWhlRotDir_enum) -> bus_creator/69
  bus_selector8/6 -> outpmodule/552(VNMM_NodeID_enum)  "<VNMM_NodeID_enum>"
  outpmodule/815(VOUTP_FACESet_enum) -> bus_creator/815
  outpmodule/190(VOUTP_RRDoorSW_flg) -> bus_creator/190
  bus_selector16/64 -> outpmodule/1046(VVMC_ADASLFCSta_enum)  "<VVMC_ADASLFCSta_enum>"
  outpmodule/741(VOUTP_AirIntenZone3MSet2_enum) -> bus_creator/741
  bus_selector4/52 -> outpmodule/409(VDDM_MCUF1NoComDTC_raw32)  "<VDDM_MCUF1NoComDTC_raw32>"
  bus_selector3/110 -> outpmodule/288(VBCM_AmbBrightnessSta5_enum)  "<VBCM_AmbBrightnessSta5_enum>"
  bus_selector16/60 -> outpmodule/1042(VVMC_TargetType_enum)  "<VVMC_TargetType_enum>"
  bus_selector3/92 -> outpmodule/270(VBCM_fUnlockSingle_flg)  "<VBCM_fUnlockSingle_flg>"
  bus_selector16/67 -> outpmodule/1049(VVMC_ADASSLIFSta_enum)  "<VVMC_ADASSLIFSta_enum>"
  outpmodule/487(VOUTP_EPBLockTODTC_raw32) -> bus_creator/487
  outpmodule/583(VOUTP_EvccAplusPwrUpReq_flg) -> bus_creator/583
  outpmodule/79(VOUTP_LFPulseCount_enum) -> bus_creator/79
  bus_selector12/96 -> outpmodule/921(VTPM_ModelVersion_raw)  "<VTPM_ModelVersion_raw>"
  outpmodule/253(VOUTP_MFRDNBrightReq_pct) -> bus_creator/253
  bus_selector3/127 -> outpmodule/305(VBCM_HBeamADB_flg)  "<VBCM_HBeamADB_flg>"
  bus_selector2/110 -> outpmodule/113(VAPM_YawRateV_flg)  "<VAPM_YawRateV_flg>"
  outpmodule/631(VOUTP_SHA4_cnt) -> bus_creator/631
  outpmodule/1067(VOUTP_FCMLDWFault_flg) -> bus_creator/1067
  bus_selector16/62 -> outpmodule/1044(VVMC_LKAHODDisplayWarning_flg)  "<VVMC_LKAHODDisplayWarning_flg>"
  outpmodule/76(VOUTP_LRPulseCountVTimeOut_flg) -> bus_creator/76
  bus_selector3/23 -> outpmodule/201(VBCM_LBeam_flg)  "<VBCM_LBeam_flg>"
  bus_selector10/39 -> outpmodule/645(VSYS_PmicBootPath_raw32)  "<VSYS_PmicBootPath_raw32>"
  bus_selector16/61 -> outpmodule/1043(VVMC_ADASSLIFSpdLim_enum)  "<VVMC_ADASSLIFSpdLim_enum>"
  bus_selector3/90 -> outpmodule/268(VBCM_LockAlarm_enum)  "<VBCM_LockAlarm_enum>"
  outpmodule/318(VOUTP_UserHeightSet_cnt) -> bus_creator/318
  bus_selector16/56 -> outpmodule/1038(VVMC_ForceLowBeam_enum)  "<VVMC_ForceLowBeam_enum>"
  outpmodule/168(VOUTP_PUIDLowPower_flg) -> bus_creator/168
  bus_selector4/131 -> outpmodule/488(VDDM_EPBUnlockTODTC_raw32)  "<VDDM_EPBUnlockTODTC_raw32>"
  bus_selector16/58 -> outpmodule/1040(VVMC_ADASWarningMsg_enum)  "<VVMC_ADASWarningMsg_enum>"
  outpmodule/8(VOUTP_ChrgPlugSta_enum) -> bus_creator/8
  bus_selector2/102 -> outpmodule/105(VAPM_YawRate_degps)  "<VAPM_YawRate_degps>"
  bus_selector16/57 -> outpmodule/1039(VVMC_ACCTakeoverReq_flg)  "<VVMC_ACCTakeoverReq_flg>"
  bus_selector2/66 -> outpmodule/69(VAPM_RRWhlRotDir_enum)  "<VAPM_RRWhlRotDir_enum>"
  bus_selector2/127 -> outpmodule/130(VAPM_EPBExtReleaseAvailTimeOut_flg)  "<VAPM_EPBExtReleaseAvailTimeOut_flg>"
  bus_selector16/79 -> outpmodule/1061(VVMC_ADASLanetypeR_enum)  "<VVMC_ADASLanetypeR_enum>"
  outpmodule/521(VOUTP_EAPS2MIN_pct) -> bus_creator/521
  outpmodule/85(VOUTP_RRPulseCount_enum) -> bus_creator/85
  bus_selector2/36 -> outpmodule/39(VAPM_USSStaFCR_flg)  "<VAPM_USSStaFCR_flg>"
  bus_selector9/39 -> outpmodule/597(VPMM_CtrlFrBMSCCUCIR_flg)  "<VPMM_CtrlFrBMSCCUCIR_flg>"
  bus_selector16/55 -> outpmodule/1037(VVMC_ACCObjDstLvl_enum)  "<VVMC_ACCObjDstLvl_enum>"
  bus_selector9/14 -> outpmodule/572(VPMM_FrMCUEnaReq_flg)  "<VPMM_FrMCUEnaReq_flg>"
  outpmodule/413(VOUTP_ESC1NoComDTC_raw32) -> bus_creator/413
  bus_selector2/78 -> outpmodule/81(VAPM_RFPulseCount_enum)  "<VAPM_RFPulseCount_enum>"
  bus_selector15/4 -> outpmodule/979(VV2L_ReqOBCExtrV2LEna_enum)  "<VV2L_ReqOBCExtrV2LEna_enum>"
  outpmodule/131(VOUTP_EPBExtApplyAvail_flg) -> bus_creator/131
  outpmodule/1004(VOUTP_ISOJerkLimit_mps3) -> bus_creator/1004
  bus_selector13/42 -> outpmodule/964(VTQD_IVIPwrLockSta_enum)  "<VTQD_IVIPwrLockSta_enum>"
  outpmodule/927(VOUTP_RrEDUAvailBrkRgnTq_Nm) -> bus_creator/927
  bus_selector16/53 -> outpmodule/1035(VVMC_ADASLDWSta_enum)  "<VVMC_ADASLDWSta_enum>"
  bus_selector16/51 -> outpmodule/1033(VVMC_LeftTurnLightReq_flg)  "<VVMC_LeftTurnLightReq_flg>"
  outpmodule/232(VOUTP_AmbLightBrightness1_enum) -> bus_creator/232
  bus_selector2/43 -> outpmodule/46(VAPM_BrkPedalPosTimeOut_flg)  "<VAPM_BrkPedalPosTimeOut_flg>"
  bus_selector16/50 -> outpmodule/1032(VVMC_RightTurnLightReq_flg)  "<VVMC_RightTurnLightReq_flg>"
  bus_selector16/52 -> outpmodule/1034(VVMC_ADASFCWSta_enum)  "<VVMC_ADASFCWSta_enum>"
  bus_selector3/80 -> outpmodule/258(VBCM_PsRWdwCtrlCmd_pct)  "<VBCM_PsRWdwCtrlCmd_pct>"
  outpmodule/37(VOUTP_USSStaFLR_flg) -> bus_creator/37
  outpmodule/203(VOUTP_RrFogLamp_flg) -> bus_creator/203
  bus_selector12/25 -> outpmodule/850(VTPM_LRPressIndi_enum)  "<VTPM_LRPressIndi_enum>"
  outpmodule/535(VOUTP_KeyAreaPTG_enum) -> bus_creator/535
  outpmodule/1071(VOUTP_CCCtrlSta_enum) -> bus_creator/1071
  bus_selector16/46 -> outpmodule/1028(VVMC_ADASShftPosnReqA_flg)  "<VVMC_ADASShftPosnReqA_flg>"
  bus_selector16/48 -> outpmodule/1030(VVMC_ADASForceIdle_flg)  "<VVMC_ADASForceIdle_flg>"
  bus_selector13/47 -> outpmodule/969(VTQD_SpdCtrlSta_flg)  "<VTQD_SpdCtrlSta_flg>"
  outpmodule/674(VOUTP_CCUACMaxLampSts_flg) -> bus_creator/674
  bus_selector16/47 -> outpmodule/1029(VVMC_ADASShftPosnReq_enum)  "<VVMC_ADASShftPosnReq_enum>"
  outpmodule/748(VOUTP_FDCFGSChStaSet457_enum) -> bus_creator/748
  outpmodule/174(VOUTP_RAPSBCMLockReq_flg) -> bus_creator/174
  bus_selector10/5 -> outpmodule/611(VSYS_CarModel2_cnt)  "<VSYS_CarModel2_cnt>"
  bus_selector16/49 -> outpmodule/1031(VVMC_HazardWarningReq_flg)  "<VVMC_HazardWarningReq_flg>"
  outpmodule/116(VOUTP_LatAccelVTimeOut_flg) -> bus_creator/116
  outpmodule/600(VOUTP_CtrlDrPwrStbA2_flg) -> bus_creator/600
  bus_selector16/74 -> outpmodule/1056(VVMC_LVDAFailinfo_flg)  "<VVMC_LVDAFailinfo_flg>"
  outpmodule/195(VOUTP_CTDCtrl_enum) -> bus_creator/195
  outpmodule/840(VOUTP_LRSensorFail_flg) -> bus_creator/840
  bus_selector16/77 -> outpmodule/1059(VVMC_ADASLFCWarnSound_enum)  "<VVMC_ADASLFCWarnSound_enum>"
  bus_selector16/44 -> outpmodule/1026(VVMC_ACCComfortBandLower_mps2)  "<VVMC_ACCComfortBandLower_mps2>"
  outpmodule/658(VOUTP_FDTWVCmd_pct) -> bus_creator/658
  outpmodule/237(VOUTP_AmbLightBrightness6_enum) -> bus_creator/237
  bus_selector16/45 -> outpmodule/1027(VVMC_ADASVehSpdLim_raw32)  "<VVMC_ADASVehSpdLim_raw32>"
  outpmodule/163(VOUTP_APSVRqEPASCtrl_flg) -> bus_creator/163
  bus_selector4/10 -> outpmodule/367(VDDM_C3CCU2RCDTC_raw32)  "<VDDM_C3CCU2RCDTC_raw32>"
  outpmodule/222(VOUTP_FrWiperH_flg) -> bus_creator/222
  bus_selector3/48 -> outpmodule/226(VBCM_AmbLightBreath1_enum)  "<VBCM_AmbLightBreath1_enum>"
  bus_selector16/42 -> outpmodule/1024(VVMC_ACCComfortBandUpper_mps2)  "<VVMC_ACCComfortBandUpper_mps2>"
  outpmodule/385(VOUTP_BMSRdyDTC_raw32) -> bus_creator/385
  bus_selector16/73 -> outpmodule/1055(VVMC_LVDAMuteSta_enum)  "<VVMC_LVDAMuteSta_enum>"
  outpmodule/730(VOUTP_fdefogSet_enum) -> bus_creator/730
  bus_selector3/167 -> outpmodule/345(VBCM_HMIKey7FuncSta_enum)  "<VBCM_HMIKey7FuncSta_enum>"
  outpmodule/926(VOUTP_FrEDUAvailBrkRgnTq_Nm) -> bus_creator/926
  bus_selector16/40 -> outpmodule/1022(VVMC_TimeGapLevel_enum)  "<VVMC_TimeGapLevel_enum>"
  bus_selector3/159 -> outpmodule/337(VBCM_AutoUnlockSta_flg)  "<VBCM_AutoUnlockSta_flg>"
  bus_selector16/39 -> outpmodule/1021(VVMC_ACCObjRelSpd_mps)  "<VVMC_ACCObjRelSpd_mps>"
  bus_selector16/32 -> outpmodule/1014(VVMC_ADASAEBReq_enum)  "<VVMC_ADASAEBReq_enum>"
  bus_selector5/6 -> outpmodule/524(VDHP_EAPS2NRM_pct)  "<VDHP_EAPS2NRM_pct>"
  bus_selector2/130 -> outpmodule/133(VAPM_EPBErrSta_enum)  "<VAPM_EPBErrSta_enum>"
  bus_selector16/31 -> outpmodule/1013(VVMC_LKATOIAct_enum)  "<VVMC_LKATOIAct_enum>"
  bus_selector4/18 -> outpmodule/375(VDDM_Lv3ErrDTC_raw32)  "<VDDM_Lv3ErrDTC_raw32>"
  outpmodule/772(VOUTP_FDCTHCREVentZStaSet2_enum) -> bus_creator/772
  bus_selector4/76 -> outpmodule/433(VDDM_FCM2NoComDTC_raw32)  "<VDDM_FCM2NoComDTC_raw32>"
  bus_selector16/36 -> outpmodule/1018(VVMC_ADASDBSReq_enum)  "<VVMC_ADASDBSReq_enum>"
  outpmodule/729(VOUTP_FootMSet_enum) -> bus_creator/729
  outpmodule/57(VOUTP_RFRawWhlSpeedV_flg) -> bus_creator/57
  bus_selector3/94 -> outpmodule/272(VBCM_AmbFunENFlash_enum)  "<VBCM_AmbFunENFlash_enum>"
  outpmodule/1084(VOUTP_ExtraMSACtrlSta_enum) -> bus_creator/1084
  bus_selector16/71 -> outpmodule/1053(VVMC_ADASLFCHandsOffWarning_enum)  "<VVMC_ADASLFCHandsOffWarning_enum>"
  bus_selector16/35 -> outpmodule/1017(VVMC_ACCVehHoldReq_flg)  "<VVMC_ACCVehHoldReq_flg>"
  bus_selector4/96 -> outpmodule/453(VDDM_ISAMalfuncDetDTC_raw32)  "<VDDM_ISAMalfuncDetDTC_raw32>"
  outpmodule/45(VOUTP_BrkPedalPos_pct) -> bus_creator/45
  bus_selector3/21 -> outpmodule/199(VBCM_DimmerEN_flg)  "<VBCM_DimmerEN_flg>"
  bus_selector8/12 -> outpmodule/558(VNMM_NetworkReq_flg)  "<VNMM_NetworkReq_flg>"
  bus_selector2/113 -> outpmodule/116(VAPM_LatAccelVTimeOut_flg)  "<VAPM_LatAccelVTimeOut_flg>"
  bus_selector16/33 -> outpmodule/1015(VVMC_ADASFaultSta_flg)  "<VVMC_ADASFaultSta_flg>"
  bus_selector6/11 -> outpmodule/535(VDKC_KeyAreaPTG_enum)  "<VDKC_KeyAreaPTG_enum>"
  bus_selector8/3 -> outpmodule/549(VNMM_Awake_enum)  "<VNMM_Awake_enum>"
  bus_selector9/8 -> outpmodule/566(VPMM_HVBatCnctReq_flg)  "<VPMM_HVBatCnctReq_flg>"
  bus_selector5/5 -> outpmodule/523(VDHP_EAPS1NRM_pct)  "<VDHP_EAPS1NRM_pct>"
  bus_selector3/117 -> outpmodule/295(VBCM_TurnSwSta_enum)  "<VBCM_TurnSwSta_enum>"
  bus_selector13/28 -> outpmodule/950(VTQD_RrRgnPermSta_flg)  "<VTQD_RrRgnPermSta_flg>"
  bus_selector16/38 -> outpmodule/1020(VVMC_ACCObjDist_m)  "<VVMC_ACCObjDist_m>"
  bus_selector8/4 -> outpmodule/550(VNMM_CSB_flg)  "<VNMM_CSB_flg>"
  bus_selector13/19 -> outpmodule/941(VTQD_FrEDUSpd_rpm)  "<VTQD_FrEDUSpd_rpm>"
  outpmodule/39(VOUTP_USSStaFCR_flg) -> bus_creator/39
  bus_selector16/34 -> outpmodule/1016(VVMC_AEBVehHoldReq_flg)  "<VVMC_AEBVehHoldReq_flg>"
  bus_selector8/2 -> outpmodule/548(VNMM_NMmTxReq_flg)  "<VNMM_NMmTxReq_flg>"
  bus_selector11/135 -> outpmodule/784(VTHC_FDCTHCLEVentYStaSet2_enum)  "<VTHC_FDCTHCLEVentYStaSet2_enum>"
  bus_selector2/118 -> outpmodule/121(VAPM_BrkSwSta_flg)  "<VAPM_BrkSwSta_flg>"
  bus_selector16/43 -> outpmodule/1025(VVMC_ACCJerkLowerLimit_mps3)  "<VVMC_ACCJerkLowerLimit_mps3>"
  outpmodule/211(VOUTP_LTurnLP_flg) -> bus_creator/211
  bus_selector8/1 -> outpmodule/547(VNMM_AllCANTxReq_flg)  "<VNMM_AllCANTxReq_flg>"
  outpmodule/957(VOUTP_RrUdcMin_V) -> bus_creator/957
  BDSC_outputs/1 -> bus_selector7/1
  outpmodule/169(VOUTP_CAASVMCReqA_flg) -> bus_creator/169
  bus_selector16/88 -> outpmodule/1070(VVMC_TimeGapCalcu_s)  "<VVMC_TimeGapCalcu_s>"
  bus_selector3/152 -> outpmodule/330(VBCM_ACCLevelMem12_enum)  "<VBCM_ACCLevelMem12_enum>"
  bus_selector11/148 -> outpmodule/797(VTHC_FDCTHCREVentYStaSet3_enum)  "<VTHC_FDCTHCREVentYStaSet3_enum>"
  bus_selector7/4 -> outpmodule/546(VDSC_DISCButtSta_flg)  "<VDSC_DISCButtSta_flg>"
  bus_selector2/56 -> outpmodule/59(VAPM_LRRawWhlSpeedV_flg)  "<VAPM_LRRawWhlSpeedV_flg>"
  outpmodule/406(VOUTP_APS1SigOoRDTC_raw32) -> bus_creator/406
  outpmodule/184(VOUTP_AntitheftSeatFlod_flg) -> bus_creator/184
  outpmodule/762(VOUTP_FDCTHCLEVentZStaSet4_enum) -> bus_creator/762
  bus_selector16/37 -> outpmodule/1019(VVMC_ADASACCSta_enum)  "<VVMC_ADASACCSta_enum>"
  outpmodule/274(VOUTP_AmbDimENFlash_enum) -> bus_creator/274
  bus_selector7/3 -> outpmodule/545(VDSC_DISCSta_enum)  "<VDSC_DISCSta_enum>"
  bus_selector2/144 -> outpmodule/147(VAPM_CAASSw_enum)  "<VAPM_CAASSw_enum>"
  bus_selector9/4 -> outpmodule/562(VPMM_PowerDownFault_enum)  "<VPMM_PowerDownFault_enum>"
  bus_selector7/2 -> outpmodule/544(VDSC_DISCTargetSpd_kph)  "<VDSC_DISCTargetSpd_kph>"
  bus_selector4/93 -> outpmodule/450(VDDM_ACCMalfuncDetDTC_raw32)  "<VDDM_ACCMalfuncDetDTC_raw32>"
  BDKC_outputs/1 -> bus_selector6/1
  outpmodule/193(VOUTP_RrChargingDoorCtrl_enum) -> bus_creator/193
  outpmodule/230(VOUTP_AmbLightBreath5_enum) -> bus_creator/230
  bus_selector11/34 -> outpmodule/683(VTHC_sigClntTHvBattIn_C)  "<VTHC_sigClntTHvBattIn_C>"
  bus_selector16/59 -> outpmodule/1041(VVMC_ADASCAMSpdLim_enum)  "<VVMC_ADASCAMSpdLim_enum>"
  outpmodule/897(VOUTP_LRPindi_enum) -> bus_creator/897
  bus_selector6/15 -> outpmodule/539(VDKC_ParkingModeCmd_enum)  "<VDKC_ParkingModeCmd_enum>"
  outpmodule/63(VOUTP_LFWhlRotDir_enum) -> bus_creator/63
  bus_selector16/70 -> outpmodule/1052(VVMC_ADASFCWMute_flg)  "<VVMC_ADASFCWMute_flg>"
  outpmodule/965(VOUTP_OPDHoldLamp_flg) -> bus_creator/965
  outpmodule/139(VOUTP_AVMparkingexcute_enum) -> bus_creator/139
  bus_selector6/18 -> outpmodule/542(VDKC_FDCDKCAllowSleep_flg)  "<VDKC_FDCDKCAllowSleep_flg>"
  outpmodule/1015(VOUTP_ADASFaultSta_flg) -> bus_creator/1015
  bus_selector16/41 -> outpmodule/1023(VVMC_ACCJerkUpperLimit_mps3)  "<VVMC_ACCJerkUpperLimit_mps3>"
  bus_selector9/9 -> outpmodule/567(VPMM_HVSysReadyToCharge_enum)  "<VPMM_HVSysReadyToCharge_enum>"
  bus_selector4/133 -> outpmodule/490(VDDM_DTCDetect_enum)  "<VDDM_DTCDetect_enum>"
  bus_selector2/96 -> outpmodule/99(VAPM_SASCAL_flg)  "<VAPM_SASCAL_flg>"
  outpmodule/148(VOUTP_CAASSwTimeOut_flg) -> bus_creator/148
  bus_selector16/72 -> outpmodule/1054(VVMC_LVDADisabled_flg)  "<VVMC_LVDADisabled_flg>"
  bus_selector3/14 -> outpmodule/192(VBCM_FrChargingDoorCtrl_enum)  "<VBCM_FrChargingDoorCtrl_enum>"
  outpmodule/719(VOUTP_FDCFGSAirIntCmd_enum) -> bus_creator/719
  outpmodule/189(VOUTP_RLDoorSW_flg) -> bus_creator/189
  bus_selector6/17 -> outpmodule/541(VDKC_KeyTypeSta_enum)  "<VDKC_KeyTypeSta_enum>"
  bus_selector7/1 -> outpmodule/543(VDSC_DISCTurn_flg)  "<VDSC_DISCTurn_flg>"
  outpmodule/859(VOUTP_RFWheelPSW_raw8) -> bus_creator/859
  outpmodule/206(VOUTP_LDRL_flg) -> bus_creator/206
  bus_selector4/140 -> outpmodule/497(VDDM_HVRlyOpFail_flg)  "<VDDM_HVRlyOpFail_flg>"
  outpmodule/775(VOUTP_FDCTHCREVentZStaSet5_enum) -> bus_creator/775
  bus_selector16/54 -> outpmodule/1036(VVMC_ADASFltWrnReq_flg)  "<VVMC_ADASFltWrnReq_flg>"
  bus_selector6/14 -> outpmodule/538(VDKC_DkeyAreaRAPSSta_enum)  "<VDKC_DkeyAreaRAPSSta_enum>"
  bus_selector16/63 -> outpmodule/1045(VVMC_LKAHODSoundWarning_flg)  "<VVMC_LKAHODSoundWarning_flg>"
  bus_selector3/141 -> outpmodule/319(VBCM_PTGUserHeight1_cnt)  "<VBCM_PTGUserHeight1_cnt>"
  bus_selector2/46 -> outpmodule/49(VAPM_RFRawWhlSpeed_kph)  "<VAPM_RFRawWhlSpeed_kph>"
  bus_selector6/16 -> outpmodule/540(VDKC_KeyNumSta_enum)  "<VDKC_KeyNumSta_enum>"
  bus_selector11/94 -> outpmodule/743(VTHC_AirIntenZone3MSet4_enum)  "<VTHC_AirIntenZone3MSet4_enum>"
